simulink model "CryoDetHcd"  (R2016b)
settings: Solver=ode45  StartTime=0.0  StopTime=1e-3  RelTol=1e-3
PreLoadFcn:
  | setup_hcd
values from neighbouring files (symbols this model uses):
  A = sqrt(0.5*erfc(x))    [setup_hcd.m]
  etaRomData = zeros(1,128)    [setup_hcd.m]
  Fadc = 614e6    (= 614000000)    [setup_hcd.m]
  freqRomData = zeros(1,128)    [setup_hcd.m]
  freqRomData1 = zeros(1,128)    [setup_hcd.m]
  freqRomData2 = zeros(1,128)    [setup_hcd.m]
  freqRomData3 = zeros(1,128)    [setup_hcd.m]
undefined symbols (not defined in the file or in its folder): AXI4, B, C, D, j, Lite
libraries: xbsIndex_r4 x2151, CryoDetLibCMB x28, hdlsllib x8, dspsigops x2, simulink x1
(part 6 of 17)

== system CryoDetHcd/DspCore/DSP/analysis_pipelined/Analysis0/channel_select1 ==
  tready : Inport
  data_valid : Inport  Port=2
  Constant : xbsIndex_r4/Constant  const=6  gui_display_data_type=Fixed-point  arith_type=Unsigned  n_bits=3  bin_pt=0  preci_type=Single  exp_width=8  frac_width=24  explicit_period=off  period=1  equ=P=C  opselect=C  inp2=PCIN>>17  opr=+  inp1=P  carry=CIN  dbl_ovrd=off  block_type=constant
  Counter : xbsIndex_r4/Counter  cnt_type=Free Running  cnt_to=Inf  operation=Up  start_count=0  cnt_by_val=1  arith_type=Unsigned  n_bits=3  bin_pt=0  load_pin=off  rst=on  en=on  explicit_period=on  period=2/Fadc  use_behavioral_HDL=off  implementation=Fabric  dbl_ovrd=off  block_type=counter
  Logical6 : xbsIndex_r4/Logical  logical_function=AND  inputs=2  en=off  latency=1  precision=Full  arith_type=Unsigned  n_bits=16  bin_pt=0  align_bp=on  dbl_ovrd=off  block_type=logical
  Relational : xbsIndex_r4/Relational  mode=a=b  op_type=Bool  en=off  latency=1  dbl_ovrd=off  block_type=relational
  tvalid : Outport
  tdata_fsel : Outport  Port=2
  t_last : Outport  Port=3
  wires:
  Logical6/1 -> Counter/2, tvalid/1
  data_valid/1 -> Logical6/2
  Counter/1 -> Relational/2, tdata_fsel/1
  tready/1 -> Logical6/1
  Relational/1 -> t_last/1
  Constant/1 -> Relational/1
  [reset] -> Counter/1

== system CryoDetHcd/DspCore/DSP/analysis_pipelined/Analysis0/scale1 ==
  note: do we saturate here or later???
  sel : Inport
  valid_i : Inport  Port=2
  In1 : Inport  Port=3
  Convert2 : xbsIndex_r4/Convert  gui_display_data_type=Boolean  arith_type=Boolean  n_bits=16  bin_pt=15  float_type=Single  exp_bits=8  fraction_bits=24  quantization=Truncate  overflow=Flag as error  en=off  latency=0  pipeline=off  dbl_ovrd=off  block_type=convert
  Delay : xbsIndex_r4/Delay  rst=off  infoeditControl=Selection of Reset will increase slice count due to use of real FFs and instead of SRLs  en=off  latency=1  reg_retiming=off  dbl_ovrd=off  block_type=delay
  Delay1 : xbsIndex_r4/Delay  rst=off  infoeditControl=Selection of Reset will increase slice count due to use of real FFs and instead of SRLs  en=off  latency=1  reg_retiming=off  dbl_ovrd=off  block_type=delay
  Delay2 : xbsIndex_r4/Delay  rst=off  infoeditControl=Selection of Reset will increase slice count due to use of real FFs and instead of SRLs  en=off  latency=1  reg_retiming=off  dbl_ovrd=off  block_type=delay
  Mux1 : xbsIndex_r4/Mux  inputs=2  en=off  latency=1  precision=User Defined  arith_type="Signed  (2's comp)"  n_bits=18  bin_pt=17  quantization=Truncate  overflow=Saturate  dbl_ovrd=off  block_type=mux
  Mux2 : xbsIndex_r4/Mux  inputs=2  en=off  latency=1  precision=User Defined  arith_type="Signed  (2's comp)"  n_bits=18  bin_pt=17  quantization=Truncate  overflow=Saturate  dbl_ovrd=off  block_type=mux
  high : xbsIndex_r4/BitBasher  bitexpr=|  display_expr=off  sr_1=im_out  arith_type1="Signed  (2's comp)"  bin_pt1=17  sr_2=re_out  arith_type2="Signed  (2's comp)"  bin_pt2=17  sr_3=indx  arith_type3=Unsigned  bin_pt3=0  sr_4=tlast  arith_type4=Unsigned  bin_pt4=0  dbl_ovrd=off  block_type=bitbasher
      | im_out ={ in[39:21] }
      | re_out = { in[18:0] }
      | indx    = { in[44:42] } 
      | tlast     = { in[45] }
  slice8 : xbsIndex_r4/BitBasher  bitexpr=|  display_expr=off  sr_1=im_out  arith_type1="Signed  (2's comp)"  bin_pt1=17  sr_2=re_out  arith_type2="Signed  (2's comp)"  bin_pt2=17  sr_3=indx  arith_type3=Unsigned  bin_pt3=0  sr_4=tlast  arith_type4=Unsigned  bin_pt4=0  dbl_ovrd=off  block_type=bitbasher
      | im_out ={ in[39:22] }
      | re_out = { in[18:1] }
      | indx    = { in[44:42] } 
      | tlast     = { in[45] }
  valid_o : Outport
  im : Outport  Port=2
  re : Outport  Port=3
  indx : Outport  Port=4
  tlast : Outport  Port=5
  wires:
  Convert2/1 -> Delay2/1
  In1/1 -> slice8/1, high/1
  high/3 -> Delay1/1
  high/4 -> Convert2/1
  high/2 -> Mux1/3
  slice8/2 -> Mux1/2
  Mux1/1 -> re/1
  high/1 -> Mux2/3
  Delay2/1 -> tlast/1
  valid_i/1 -> Delay/1
  slice8/1 -> Mux2/2
  Delay/1 -> valid_o/1
  Mux2/1 -> im/1
  Delay1/1 -> indx/1
  sel/1 -> Mux2/1, Mux1/1

== system CryoDetHcd/DspCore/DSP/analysis_pipelined/Analysis0/scale2 ==
  note: do we saturate here or later???
  sel : Inport
  valid_i : Inport  Port=2
  In1 : Inport  Port=3
  Delay : xbsIndex_r4/Delay  rst=off  infoeditControl=Selection of Reset will increase slice count due to use of real FFs and instead of SRLs  en=off  latency=1  reg_retiming=off  dbl_ovrd=off  block_type=delay
  Delay1 : xbsIndex_r4/Delay  rst=off  infoeditControl=Selection of Reset will increase slice count due to use of real FFs and instead of SRLs  en=off  latency=1  reg_retiming=off  dbl_ovrd=off  block_type=delay
  Mux1 : xbsIndex_r4/Mux  inputs=2  en=off  latency=1  precision=User Defined  arith_type="Signed  (2's comp)"  n_bits=18  bin_pt=17  quantization=Truncate  overflow=Saturate  dbl_ovrd=off  block_type=mux
  Mux2 : xbsIndex_r4/Mux  inputs=2  en=off  latency=1  precision=User Defined  arith_type="Signed  (2's comp)"  n_bits=18  bin_pt=17  quantization=Truncate  overflow=Saturate  dbl_ovrd=off  block_type=mux
  high : xbsIndex_r4/BitBasher  bitexpr=|  display_expr=off  sr_1=re  arith_type1="Signed  (2's comp)"  bin_pt1=17  sr_2=im  arith_type2="Signed  (2's comp)"  bin_pt2=17  sr_3=indx  arith_type3=Unsigned  bin_pt3=0  sr_4=4  arith_type4=Unsigned  bin_pt4=0  dbl_ovrd=off  block_type=bitbasher
      | re={in[18:0]}
      | im={in[44:26]}
      | indx ={in[54:52]}
  nominal : xbsIndex_r4/BitBasher  bitexpr=|  display_expr=off  sr_1=re  arith_type1="Signed  (2's comp)"  bin_pt1=17  sr_2=im  arith_type2="Signed  (2's comp)"  bin_pt2=17  sr_3=indx  arith_type3=Unsigned  bin_pt3=0  sr_4=4  arith_type4=Unsigned  bin_pt4=0  dbl_ovrd=off  block_type=bitbasher
      | re={in[18:1]}
      | im={in[44:27]}
      | indx ={in[54:52]}
  valid_o : Outport
  re : Outport  Port=2
  im : Outport  Port=3
  indx : Outport  Port=4
  wires:
  sel/1 -> Mux1/1, Mux2/1
  Delay1/1 -> indx/1
  Delay/1 -> valid_o/1
  valid_i/1 -> Delay/1
  In1/1 -> nominal/1, high/1
  Mux2/1 -> re/1
  Mux1/1 -> im/1
  high/3 -> Delay1/1
  high/2 -> Mux1/3
  high/1 -> Mux2/3
  nominal/1 -> Mux2/2
  nominal/2 -> Mux1/2

== system CryoDetHcd/DspCore/DSP/analysis_pipelined/Analysis0/scale3 ==
  note: do we saturate here or later???
  sel : Inport
  valid_i : Inport  Port=2
  In1 : Inport  Port=3
  Delay : xbsIndex_r4/Delay  rst=off  infoeditControl=Selection of Reset will increase slice count due to use of real FFs and instead of SRLs  en=off  latency=1  reg_retiming=off  dbl_ovrd=off  block_type=delay
  Delay1 : xbsIndex_r4/Delay  rst=off  infoeditControl=Selection of Reset will increase slice count due to use of real FFs and instead of SRLs  en=off  latency=1  reg_retiming=off  dbl_ovrd=off  block_type=delay
  Mux1 : xbsIndex_r4/Mux  inputs=2  en=off  latency=1  precision=User Defined  arith_type="Signed  (2's comp)"  n_bits=18  bin_pt=17  quantization=Truncate  overflow=Saturate  dbl_ovrd=off  block_type=mux
  Mux2 : xbsIndex_r4/Mux  inputs=2  en=off  latency=1  precision=User Defined  arith_type="Signed  (2's comp)"  n_bits=18  bin_pt=17  quantization=Truncate  overflow=Saturate  dbl_ovrd=off  block_type=mux
  high : xbsIndex_r4/BitBasher  bitexpr=|  display_expr=off  sr_1=re  arith_type1="Signed  (2's comp)"  bin_pt1=17  sr_2=im  arith_type2="Signed  (2's comp)"  bin_pt2=17  sr_3=indx  arith_type3=Unsigned  bin_pt3=0  sr_4=4  arith_type4=Unsigned  bin_pt4=0  dbl_ovrd=off  block_type=bitbasher
      | re={in[18:0]}
      | im={in[44:26]}
      | indx ={in[54:52]}
  nominal : xbsIndex_r4/BitBasher  bitexpr=|  display_expr=off  sr_1=re  arith_type1="Signed  (2's comp)"  bin_pt1=17  sr_2=im  arith_type2="Signed  (2's comp)"  bin_pt2=17  sr_3=indx  arith_type3=Unsigned  bin_pt3=0  sr_4=4  arith_type4=Unsigned  bin_pt4=0  dbl_ovrd=off  block_type=bitbasher
      | re={in[18:1]}
      | im={in[44:27]}
      | indx ={in[54:52]}
  valid_o : Outport
  re : Outport  Port=2
  im : Outport  Port=3
  indx : Outport  Port=4
  wires:
  nominal/2 -> Mux1/2
  nominal/1 -> Mux2/2
  high/1 -> Mux2/3
  high/2 -> Mux1/3
  high/3 -> Delay1/1
  Mux1/1 -> im/1
  Mux2/1 -> re/1
  In1/1 -> high/1, nominal/1
  valid_i/1 -> Delay/1
  Delay/1 -> valid_o/1
  Delay1/1 -> indx/1
  sel/1 -> Mux2/1, Mux1/1

== system CryoDetHcd/DspCore/DSP/analysis_pipelined/Analysis0/scale4 ==
  note: do we saturate here or later???
  sel : Inport
  valid_i : Inport  Port=2
  In1 : Inport  Port=3
  Convert2 : xbsIndex_r4/Convert  gui_display_data_type=Boolean  arith_type=Boolean  n_bits=16  bin_pt=15  float_type=Single  exp_bits=8  fraction_bits=24  quantization=Truncate  overflow=Flag as error  en=off  latency=0  pipeline=off  dbl_ovrd=off  block_type=convert
  Delay : xbsIndex_r4/Delay  rst=off  infoeditControl=Selection of Reset will increase slice count due to use of real FFs and instead of SRLs  en=off  latency=1  reg_retiming=off  dbl_ovrd=off  block_type=delay
  Delay1 : xbsIndex_r4/Delay  rst=off  infoeditControl=Selection of Reset will increase slice count due to use of real FFs and instead of SRLs  en=off  latency=1  reg_retiming=off  dbl_ovrd=off  block_type=delay
  Delay2 : xbsIndex_r4/Delay  rst=off  infoeditControl=Selection of Reset will increase slice count due to use of real FFs and instead of SRLs  en=off  latency=1  reg_retiming=off  dbl_ovrd=off  block_type=delay
  Mux1 : xbsIndex_r4/Mux  inputs=2  en=off  latency=1  precision=User Defined  arith_type="Signed  (2's comp)"  n_bits=18  bin_pt=17  quantization=Truncate  overflow=Saturate  dbl_ovrd=off  block_type=mux
  Mux2 : xbsIndex_r4/Mux  inputs=2  en=off  latency=1  precision=User Defined  arith_type="Signed  (2's comp)"  n_bits=18  bin_pt=17  quantization=Truncate  overflow=Saturate  dbl_ovrd=off  block_type=mux
  high : xbsIndex_r4/BitBasher  bitexpr=|  display_expr=off  sr_1=im_out  arith_type1="Signed  (2's comp)"  bin_pt1=17  sr_2=re_out  arith_type2="Signed  (2's comp)"  bin_pt2=17  sr_3=indx  arith_type3=Unsigned  bin_pt3=0  sr_4=tlast  arith_type4=Unsigned  bin_pt4=0  dbl_ovrd=off  block_type=bitbasher
      | im_out ={ in[39:21] }
      | re_out = { in[18:0] }
      | indx    = { in[44:42] } 
      | tlast     = { in[45] }
  slice8 : xbsIndex_r4/BitBasher  bitexpr=|  display_expr=off  sr_1=im_out  arith_type1="Signed  (2's comp)"  bin_pt1=17  sr_2=re_out  arith_type2="Signed  (2's comp)"  bin_pt2=17  sr_3=indx  arith_type3=Unsigned  bin_pt3=0  sr_4=tlast  arith_type4=Unsigned  bin_pt4=0  dbl_ovrd=off  block_type=bitbasher
      | im_out ={ in[39:22] }
      | re_out = { in[18:1] }
      | indx    = { in[44:42] } 
      | tlast     = { in[45] }
  valid_o : Outport
  im : Outport  Port=2
  re : Outport  Port=3
  indx : Outport  Port=4
  tlast : Outport  Port=5
  wires:
  sel/1 -> Mux1/1, Mux2/1
  Delay1/1 -> indx/1
  Mux2/1 -> im/1
  Delay/1 -> valid_o/1
  slice8/1 -> Mux2/2
  valid_i/1 -> Delay/1
  Delay2/1 -> tlast/1
  high/1 -> Mux2/3
  Mux1/1 -> re/1
  slice8/2 -> Mux1/2
  high/2 -> Mux1/3
  high/4 -> Convert2/1
  high/3 -> Delay1/1
  In1/1 -> high/1, slice8/1
  Convert2/1 -> Delay2/1

== system CryoDetHcd/DspCore/DSP/analysis_pipelined/Analysis1/channel_select1 ==
  tready : Inport
  data_valid : Inport  Port=2
  Constant : xbsIndex_r4/Constant  const=6  gui_display_data_type=Fixed-point  arith_type=Unsigned  n_bits=3  bin_pt=0  preci_type=Single  exp_width=8  frac_width=24  explicit_period=off  period=1  equ=P=C  opselect=C  inp2=PCIN>>17  opr=+  inp1=P  carry=CIN  dbl_ovrd=off  block_type=constant
  Counter : xbsIndex_r4/Counter  cnt_type=Free Running  cnt_to=Inf  operation=Up  start_count=0  cnt_by_val=1  arith_type=Unsigned  n_bits=3  bin_pt=0  load_pin=off  rst=on  en=on  explicit_period=on  period=2/Fadc  use_behavioral_HDL=off  implementation=Fabric  dbl_ovrd=off  block_type=counter
  Logical6 : xbsIndex_r4/Logical  logical_function=AND  inputs=2  en=off  latency=1  precision=Full  arith_type=Unsigned  n_bits=16  bin_pt=0  align_bp=on  dbl_ovrd=off  block_type=logical
  Relational : xbsIndex_r4/Relational  mode=a=b  op_type=Bool  en=off  latency=1  dbl_ovrd=off  block_type=relational
  tvalid : Outport
  tdata_fsel : Outport  Port=2
  t_last : Outport  Port=3
  wires:
  [reset] -> Counter/1
  Constant/1 -> Relational/1
  Relational/1 -> t_last/1
  tready/1 -> Logical6/1
  Counter/1 -> tdata_fsel/1, Relational/2
  data_valid/1 -> Logical6/2
  Logical6/1 -> tvalid/1, Counter/2

== system CryoDetHcd/DspCore/DSP/analysis_pipelined/Analysis1/scale1 ==
  note: do we saturate here or later???
  sel : Inport
  valid_i : Inport  Port=2
  In1 : Inport  Port=3
  Convert2 : xbsIndex_r4/Convert  gui_display_data_type=Boolean  arith_type=Boolean  n_bits=16  bin_pt=15  float_type=Single  exp_bits=8  fraction_bits=24  quantization=Truncate  overflow=Flag as error  en=off  latency=0  pipeline=off  dbl_ovrd=off  block_type=convert
  Delay : xbsIndex_r4/Delay  rst=off  infoeditControl=Selection of Reset will increase slice count due to use of real FFs and instead of SRLs  en=off  latency=1  reg_retiming=off  dbl_ovrd=off  block_type=delay
  Delay1 : xbsIndex_r4/Delay  rst=off  infoeditControl=Selection of Reset will increase slice count due to use of real FFs and instead of SRLs  en=off  latency=1  reg_retiming=off  dbl_ovrd=off  block_type=delay
  Delay2 : xbsIndex_r4/Delay  rst=off  infoeditControl=Selection of Reset will increase slice count due to use of real FFs and instead of SRLs  en=off  latency=1  reg_retiming=off  dbl_ovrd=off  block_type=delay
  Mux1 : xbsIndex_r4/Mux  inputs=2  en=off  latency=1  precision=User Defined  arith_type="Signed  (2's comp)"  n_bits=18  bin_pt=17  quantization=Truncate  overflow=Saturate  dbl_ovrd=off  block_type=mux
  Mux2 : xbsIndex_r4/Mux  inputs=2  en=off  latency=1  precision=User Defined  arith_type="Signed  (2's comp)"  n_bits=18  bin_pt=17  quantization=Truncate  overflow=Saturate  dbl_ovrd=off  block_type=mux
  high : xbsIndex_r4/BitBasher  bitexpr=|  display_expr=off  sr_1=im_out  arith_type1="Signed  (2's comp)"  bin_pt1=17  sr_2=re_out  arith_type2="Signed  (2's comp)"  bin_pt2=17  sr_3=indx  arith_type3=Unsigned  bin_pt3=0  sr_4=tlast  arith_type4=Unsigned  bin_pt4=0  dbl_ovrd=off  block_type=bitbasher
      | im_out ={ in[39:21] }
      | re_out = { in[18:0] }
      | indx    = { in[44:42] } 
      | tlast     = { in[45] }
  slice8 : xbsIndex_r4/BitBasher  bitexpr=|  display_expr=off  sr_1=im_out  arith_type1="Signed  (2's comp)"  bin_pt1=17  sr_2=re_out  arith_type2="Signed  (2's comp)"  bin_pt2=17  sr_3=indx  arith_type3=Unsigned  bin_pt3=0  sr_4=tlast  arith_type4=Unsigned  bin_pt4=0  dbl_ovrd=off  block_type=bitbasher
      | im_out ={ in[39:22] }
      | re_out = { in[18:1] }
      | indx    = { in[44:42] } 
      | tlast     = { in[45] }
  valid_o : Outport
  im : Outport  Port=2
  re : Outport  Port=3
  indx : Outport  Port=4
  tlast : Outport  Port=5
  wires:
  sel/1 -> Mux1/1, Mux2/1
  Delay1/1 -> indx/1
  Mux2/1 -> im/1
  Delay/1 -> valid_o/1
  slice8/1 -> Mux2/2
  valid_i/1 -> Delay/1
  Delay2/1 -> tlast/1
  high/1 -> Mux2/3
  Mux1/1 -> re/1
  slice8/2 -> Mux1/2
  high/2 -> Mux1/3
  high/4 -> Convert2/1
  high/3 -> Delay1/1
  In1/1 -> high/1, slice8/1
  Convert2/1 -> Delay2/1

== system CryoDetHcd/DspCore/DSP/analysis_pipelined/Analysis1/scale2 ==
  note: do we saturate here or later???
  sel : Inport
  valid_i : Inport  Port=2
  In1 : Inport  Port=3
  Delay : xbsIndex_r4/Delay  rst=off  infoeditControl=Selection of Reset will increase slice count due to use of real FFs and instead of SRLs  en=off  latency=1  reg_retiming=off  dbl_ovrd=off  block_type=delay
  Delay1 : xbsIndex_r4/Delay  rst=off  infoeditControl=Selection of Reset will increase slice count due to use of real FFs and instead of SRLs  en=off  latency=1  reg_retiming=off  dbl_ovrd=off  block_type=delay
  Mux1 : xbsIndex_r4/Mux  inputs=2  en=off  latency=1  precision=User Defined  arith_type="Signed  (2's comp)"  n_bits=18  bin_pt=17  quantization=Truncate  overflow=Saturate  dbl_ovrd=off  block_type=mux
  Mux2 : xbsIndex_r4/Mux  inputs=2  en=off  latency=1  precision=User Defined  arith_type="Signed  (2's comp)"  n_bits=18  bin_pt=17  quantization=Truncate  overflow=Saturate  dbl_ovrd=off  block_type=mux
  high : xbsIndex_r4/BitBasher  bitexpr=|  display_expr=off  sr_1=re  arith_type1="Signed  (2's comp)"  bin_pt1=17  sr_2=im  arith_type2="Signed  (2's comp)"  bin_pt2=17  sr_3=indx  arith_type3=Unsigned  bin_pt3=0  sr_4=4  arith_type4=Unsigned  bin_pt4=0  dbl_ovrd=off  block_type=bitbasher
      | re={in[18:0]}
      | im={in[44:26]}
      | indx ={in[54:52]}
  nominal : xbsIndex_r4/BitBasher  bitexpr=|  display_expr=off  sr_1=re  arith_type1="Signed  (2's comp)"  bin_pt1=17  sr_2=im  arith_type2="Signed  (2's comp)"  bin_pt2=17  sr_3=indx  arith_type3=Unsigned  bin_pt3=0  sr_4=4  arith_type4=Unsigned  bin_pt4=0  dbl_ovrd=off  block_type=bitbasher
      | re={in[18:1]}
      | im={in[44:27]}
      | indx ={in[54:52]}
  valid_o : Outport
  re : Outport  Port=2
  im : Outport  Port=3
  indx : Outport  Port=4
  wires:
  nominal/2 -> Mux1/2
  nominal/1 -> Mux2/2
  high/1 -> Mux2/3
  high/2 -> Mux1/3
  high/3 -> Delay1/1
  Mux1/1 -> im/1
  Mux2/1 -> re/1
  In1/1 -> high/1, nominal/1
  valid_i/1 -> Delay/1
  Delay/1 -> valid_o/1
  Delay1/1 -> indx/1
  sel/1 -> Mux2/1, Mux1/1

== system CryoDetHcd/DspCore/DSP/analysis_pipelined/Analysis1/scale3 ==
  note: do we saturate here or later???
  sel : Inport
  valid_i : Inport  Port=2
  In1 : Inport  Port=3
  Delay : xbsIndex_r4/Delay  rst=off  infoeditControl=Selection of Reset will increase slice count due to use of real FFs and instead of SRLs  en=off  latency=1  reg_retiming=off  dbl_ovrd=off  block_type=delay
  Delay1 : xbsIndex_r4/Delay  rst=off  infoeditControl=Selection of Reset will increase slice count due to use of real FFs and instead of SRLs  en=off  latency=1  reg_retiming=off  dbl_ovrd=off  block_type=delay
  Mux1 : xbsIndex_r4/Mux  inputs=2  en=off  latency=1  precision=User Defined  arith_type="Signed  (2's comp)"  n_bits=18  bin_pt=17  quantization=Truncate  overflow=Saturate  dbl_ovrd=off  block_type=mux
  Mux2 : xbsIndex_r4/Mux  inputs=2  en=off  latency=1  precision=User Defined  arith_type="Signed  (2's comp)"  n_bits=18  bin_pt=17  quantization=Truncate  overflow=Saturate  dbl_ovrd=off  block_type=mux
  high : xbsIndex_r4/BitBasher  bitexpr=|  display_expr=off  sr_1=re  arith_type1="Signed  (2's comp)"  bin_pt1=17  sr_2=im  arith_type2="Signed  (2's comp)"  bin_pt2=17  sr_3=indx  arith_type3=Unsigned  bin_pt3=0  sr_4=4  arith_type4=Unsigned  bin_pt4=0  dbl_ovrd=off  block_type=bitbasher
      | re={in[18:0]}
      | im={in[44:26]}
      | indx ={in[54:52]}
  nominal : xbsIndex_r4/BitBasher  bitexpr=|  display_expr=off  sr_1=re  arith_type1="Signed  (2's comp)"  bin_pt1=17  sr_2=im  arith_type2="Signed  (2's comp)"  bin_pt2=17  sr_3=indx  arith_type3=Unsigned  bin_pt3=0  sr_4=4  arith_type4=Unsigned  bin_pt4=0  dbl_ovrd=off  block_type=bitbasher
      | re={in[18:1]}
      | im={in[44:27]}
      | indx ={in[54:52]}
  valid_o : Outport
  re : Outport  Port=2
  im : Outport  Port=3
  indx : Outport  Port=4
  wires:
  sel/1 -> Mux1/1, Mux2/1
  Delay1/1 -> indx/1
  Delay/1 -> valid_o/1
  valid_i/1 -> Delay/1
  In1/1 -> nominal/1, high/1
  Mux2/1 -> re/1
  Mux1/1 -> im/1
  high/3 -> Delay1/1
  high/2 -> Mux1/3
  high/1 -> Mux2/3
  nominal/1 -> Mux2/2
  nominal/2 -> Mux1/2

== system CryoDetHcd/DspCore/DSP/analysis_pipelined/Analysis1/scale4 ==
  note: do we saturate here or later???
  sel : Inport
  valid_i : Inport  Port=2
  In1 : Inport  Port=3
  Convert2 : xbsIndex_r4/Convert  gui_display_data_type=Boolean  arith_type=Boolean  n_bits=16  bin_pt=15  float_type=Single  exp_bits=8  fraction_bits=24  quantization=Truncate  overflow=Flag as error  en=off  latency=0  pipeline=off  dbl_ovrd=off  block_type=convert
  Delay : xbsIndex_r4/Delay  rst=off  infoeditControl=Selection of Reset will increase slice count due to use of real FFs and instead of SRLs  en=off  latency=1  reg_retiming=off  dbl_ovrd=off  block_type=delay
  Delay1 : xbsIndex_r4/Delay  rst=off  infoeditControl=Selection of Reset will increase slice count due to use of real FFs and instead of SRLs  en=off  latency=1  reg_retiming=off  dbl_ovrd=off  block_type=delay
  Delay2 : xbsIndex_r4/Delay  rst=off  infoeditControl=Selection of Reset will increase slice count due to use of real FFs and instead of SRLs  en=off  latency=1  reg_retiming=off  dbl_ovrd=off  block_type=delay
  Mux1 : xbsIndex_r4/Mux  inputs=2  en=off  latency=1  precision=User Defined  arith_type="Signed  (2's comp)"  n_bits=18  bin_pt=17  quantization=Truncate  overflow=Saturate  dbl_ovrd=off  block_type=mux
  Mux2 : xbsIndex_r4/Mux  inputs=2  en=off  latency=1  precision=User Defined  arith_type="Signed  (2's comp)"  n_bits=18  bin_pt=17  quantization=Truncate  overflow=Saturate  dbl_ovrd=off  block_type=mux
  high : xbsIndex_r4/BitBasher  bitexpr=|  display_expr=off  sr_1=im_out  arith_type1="Signed  (2's comp)"  bin_pt1=17  sr_2=re_out  arith_type2="Signed  (2's comp)"  bin_pt2=17  sr_3=indx  arith_type3=Unsigned  bin_pt3=0  sr_4=tlast  arith_type4=Unsigned  bin_pt4=0  dbl_ovrd=off  block_type=bitbasher
      | im_out ={ in[39:21] }
      | re_out = { in[18:0] }
      | indx    = { in[44:42] } 
      | tlast     = { in[45] }
  slice8 : xbsIndex_r4/BitBasher  bitexpr=|  display_expr=off  sr_1=im_out  arith_type1="Signed  (2's comp)"  bin_pt1=17  sr_2=re_out  arith_type2="Signed  (2's comp)"  bin_pt2=17  sr_3=indx  arith_type3=Unsigned  bin_pt3=0  sr_4=tlast  arith_type4=Unsigned  bin_pt4=0  dbl_ovrd=off  block_type=bitbasher
      | im_out ={ in[39:22] }
      | re_out = { in[18:1] }
      | indx    = { in[44:42] } 
      | tlast     = { in[45] }
  valid_o : Outport
  im : Outport  Port=2
  re : Outport  Port=3
  indx : Outport  Port=4
  tlast : Outport  Port=5
  wires:
  Convert2/1 -> Delay2/1
  In1/1 -> slice8/1, high/1
  high/3 -> Delay1/1
  high/4 -> Convert2/1
  high/2 -> Mux1/3
  slice8/2 -> Mux1/2
  Mux1/1 -> re/1
  high/1 -> Mux2/3
  Delay2/1 -> tlast/1
  valid_i/1 -> Delay/1
  slice8/1 -> Mux2/2
  Delay/1 -> valid_o/1
  Mux2/1 -> im/1
  Delay1/1 -> indx/1
  sel/1 -> Mux2/1, Mux1/1

== system CryoDetHcd/DspCore/DSP/channel_processor/channel_processor_x1/Enabled Subsystem ==
  In1 : Inport
  In2 : Inport  Port=2
  Enable : EnablePort
  Buffer : Buffer  N=8  TreatMby1Signals=One channel  OutputFrames=off
  Buffer1 : Buffer  N=8  TreatMby1Signals=One channel  OutputFrames=off
  Out1 : Outport
  Out2 : Outport  Port=2
  wires:
  In1/1 -> Buffer/1
  Buffer/1 -> Out1/1
  In2/1 -> Buffer1/1
  Buffer1/1 -> Out2/1

== system CryoDetHcd/DspCore/DSP/channel_processor/channel_processor_x1/IQ_status_sel ==
  sel : Inport
  Q : Inport  Port=2
  I : Inport  Port=3
  ch : Inport  Port=4
  BitBasher : xbsIndex_r4/BitBasher  bitexpr=out = {I,Q}  display_expr=off  sr_1=out  arith_type1=Unsigned  bin_pt1=0  sr_2=2  arith_type2=Unsigned  bin_pt2=0  sr_3=3  arith_type3=Unsigned  bin_pt3=0  sr_4=4  arith_type4=Unsigned  bin_pt4=0  dbl_ovrd=off  block_type=bitbasher
  Convert : xbsIndex_r4/Convert  gui_display_data_type=Fixed-point  arith_type="Signed  (2's comp)"  n_bits=16  bin_pt=15  float_type=Single  exp_bits=8  fraction_bits=24  quantization=Truncate  overflow=Wrap  en=off  latency=1  pipeline=off  dbl_ovrd=off  block_type=convert
  Convert1 : xbsIndex_r4/Convert  gui_display_data_type=Fixed-point  arith_type="Signed  (2's comp)"  n_bits=16  bin_pt=15  float_type=Single  exp_bits=8  fraction_bits=24  quantization=Truncate  overflow=Wrap  en=off  latency=1  pipeline=off  dbl_ovrd=off  block_type=convert
  Register2 : xbsIndex_r4/Register  init=0  rst=off  en=on  dbl_ovrd=off  block_type=register
  Relational : xbsIndex_r4/Relational  mode=a=b  op_type=Bool  en=off  latency=1  dbl_ovrd=off  block_type=relational
  IQ_status_r : Outport
  wires:
  I/1 -> Convert1/1
  Q/1 -> Convert/1
  Convert1/1 -> BitBasher/2
  ch/1 -> Relational/2
  sel/1 -> Relational/1
  Convert/1 -> BitBasher/1
  BitBasher/1 -> Register2/1
  Register2/1 -> IQ_status_r/1
  Relational/1 -> Register2/2

== system CryoDetHcd/DspCore/DSP/channel_processor/channel_processor_x1/config2_r ==
  In1 : Inport
  BitBasher : xbsIndex_r4/BitBasher  bitexpr=|  display_expr=off  sr_1=ref_delay  arith_type1=Unsigned  bin_pt1=0  sr_2=tone_scale_sel  arith_type2=Unsigned  bin_pt2=0  sr_3=fb_enable  arith_type3=Unsigned  bin_pt3=0  sr_4=fb_polarity  arith_type4=Unsigned  bin_pt4=0  dbl_ovrd=off  block_type=bitbasher
      | ref_delay = {in[2:0]}
      | tone_scale_sel = {in[4:3]}
      | fb_enable = {in[5]}
      | fb_polarity = {in[6]}
  BitBasher1 : xbsIndex_r4/BitBasher  bitexpr=|  display_expr=off  sr_1=iq_swap_sel  arith_type1=Unsigned  bin_pt1=0  sr_2=iq_band_sel  arith_type2=Unsigned  bin_pt2=0  sr_3=iq_ch_sel  arith_type3=Unsigned  bin_pt3=0  sr_4=analysis_iq_ch_sel  arith_type4=Unsigned  bin_pt4=0  dbl_ovrd=off  block_type=bitbasher
      | iq_swap_sel = {in[7]}
      | iq_band_sel = {in[16:15]}
      | iq_ch_sel = {in[14:8]}
      | analysis_iq_ch_sel={in[17:15]}
  ref_delay : Outport
  tone_scale_sel : Outport  Port=2
  fb_enable : Outport  Port=3
  fb_polarity : Outport  Port=4
  iq_swap_sel : Outport  Port=5
  iq_band_sel : Outport  Port=6
  iq_ch_sel : Outport  Port=7
  analysis_iq_sel : Outport  Port=8
  wires:
  BitBasher1/3 -> iq_ch_sel/1
  BitBasher1/2 -> iq_band_sel/1
  BitBasher1/1 -> iq_swap_sel/1
  BitBasher/4 -> fb_polarity/1
  BitBasher/3 -> fb_enable/1
  BitBasher/2 -> tone_scale_sel/1
  BitBasher/1 -> ref_delay/1
  In1/1 -> BitBasher/1, BitBasher1/1
  BitBasher1/4 -> analysis_iq_sel/1

== system CryoDetHcd/DspCore/DSP/channel_processor/channel_processor_x1/config3_r1 ==
  In1 : Inport
  BitBasher1 : xbsIndex_r4/BitBasher  bitexpr=|  display_expr=off  sr_1=fb_gain  arith_type1=Unsigned  bin_pt1=14  sr_2=fb_limit  arith_type2=Unsigned  bin_pt2=16  sr_3=ref_delay  arith_type3=Unsigned  bin_pt3=0  sr_4=4  arith_type4=Unsigned  bin_pt4=0  dbl_ovrd=off  block_type=bitbasher
      | fb_gain = {in[15:0]}
      | fb_limit = {in[31:16]}
  Negate : xbsIndex_r4/Negate  precision=User Defined  arith_type=Unsigned  n_bits=16  bin_pt=15  quantization=Truncate  overflow=Wrap  en=off  latency=2  dbl_ovrd=off  block_type=negate
  fb_gain : Outport
  fb_limit_hi : Outport  Port=2
  fb_limit_lo : Outport  Port=3
  wires:
  BitBasher1/2 -> Negate/1, fb_limit_hi/1
  In1/1 -> BitBasher1/1
  BitBasher1/1 -> fb_gain/1
  Negate/1 -> fb_limit_lo/1

== system CryoDetHcd/DspCore/DSP/channel_processor/channel_processor_x1/scale1 ==
  In1 : Inport
  Bit Slice : hdlsllib/HDL Operations/Bit Slice  lidx=15  ridx=0
  Bit Slice1 : hdlsllib/HDL Operations/Bit Slice  lidx=31  ridx=16
  Data Type Conversion : DataTypeConversion  OutDataTypeStr=int16  ConvertRealWorld=Stored Integer (SI)
  Data Type Conversion1 : DataTypeConversion  OutDataTypeStr=int16  ConvertRealWorld=Stored Integer (SI)
  Q : Outport
  I : Outport  Port=2
  wires:
  In1/1 -> Bit Slice1/1, Bit Slice/1
  Bit Slice/1 -> Data Type Conversion/1
  Data Type Conversion1/1 -> Q/1
  Bit Slice1/1 -> Data Type Conversion1/1
  Data Type Conversion/1 -> I/1

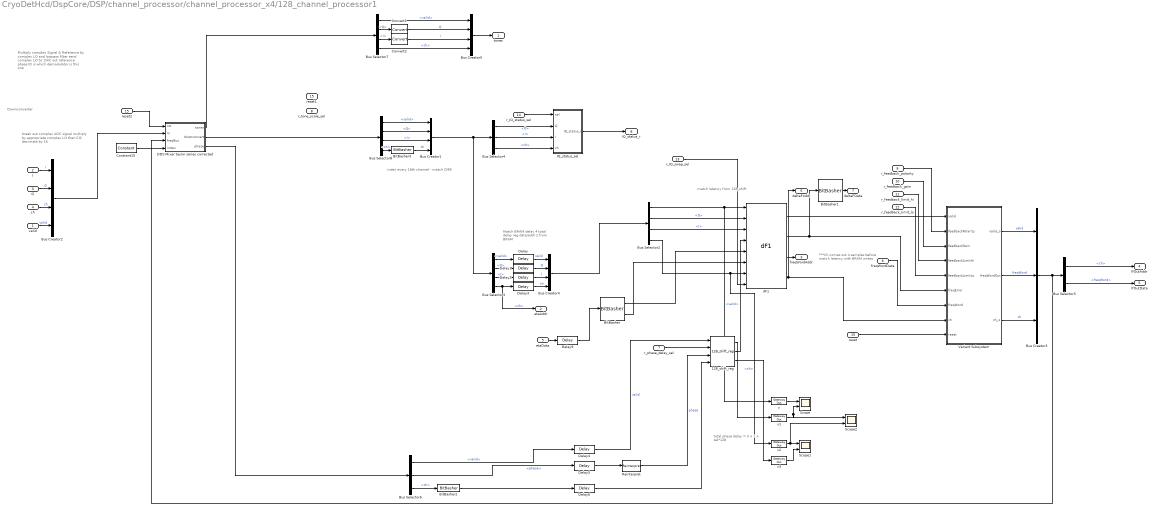
== system CryoDetHcd/DspCore/DSP/channel_processor/channel_processor_x4/128_channel_processor1 ==
  note: ***Ch comes out 4 samples before
      | match latency with BRAM writes
  note: total phase delay =
      | 3 + 1 + sel*128
  note: match latency from 128_shift
  note: Match BRAM delay
      | 4 total delay
      |    reg data/addr
      |    2 from BRAM
  note: break out complex ADC signal
      | multiply by appropriate complex LO
      | then CIC decimate by 16
  note: Multiply complex Signal & Reference
      | by complex LO and lowpass filter
      | send complex LO to:
      | 	DAC out
      | 	reference phase
      | ID is which demodulator is this one
  note: Downconverter
  note: index every 16th channel - match CMB
  valid : Inport
  I : Inport  Port=2
  Q : Inport  Port=3
  ch : Inport  Port=4
  etaData : Inport  Port=5
  freqWordData : Inport  Port=6
  r_phase_delay_sel : Inport  Port=7
  r_tone_scale_sel : Inport  Port=8
  r_feedback_polarity : Inport  Port=9
  r_feedback_gain : Inport  Port=10
  r_feedback_limit_hi : Inport  Port=11
  r_feedback_limit_lo : Inport  Port=12
  r_IQ_swap_sel : Inport  Port=13
  r_IQ_status_sel : Inport  Port=14
  reset : Inport  Port=15
  128_shift_reg : CryoDetLibCMB/128_shift_reg
  BitBasher : xbsIndex_r4/BitBasher  bitexpr=|  display_expr=off  sr_1=etaPhase  arith_type1="Signed  (2's comp)"  bin_pt1=15  sr_2=etaMag  arith_type2="Signed  (2's comp)"  bin_pt2=10  sr_3=3  arith_type3=Unsigned  bin_pt3=0  sr_4=4  arith_type4=Unsigned  bin_pt4=0  dbl_ovrd=off  block_type=bitbasher
      | etaPhase = {in[31:16]}
      | etaMag = {in[15:0]}
  BitBasher1 : xbsIndex_r4/BitBasher  bitexpr=deltaF = {8'b0, in[23:0]}  display_expr=off  sr_1=deltaF  arith_type1="Signed  (2's comp)"  bin_pt1=15  sr_2=etaMag  arith_type2="Signed  (2's comp)"  bin_pt2=10  sr_3=3  arith_type3=Unsigned  bin_pt3=0  sr_4=4  arith_type4=Unsigned  bin_pt4=0  dbl_ovrd=off  block_type=bitbasher
  BitBasher2 : xbsIndex_r4/BitBasher  bitexpr=out = {in, 4'b0000}  display_expr=off  sr_1=out  arith_type1=Unsigned  bin_pt1=0  sr_2=2  arith_type2=Unsigned  bin_pt2=0  sr_3=3  arith_type3=Unsigned  bin_pt3=0  sr_4=4  arith_type4=Unsigned  bin_pt4=0  dbl_ovrd=off  block_type=bitbasher
  BitBasher3 : xbsIndex_r4/BitBasher  bitexpr=out = {in, 4'b0000}  display_expr=off  sr_1=out  arith_type1=Unsigned  bin_pt1=0  sr_2=2  arith_type2=Unsigned  bin_pt2=0  sr_3=3  arith_type3=Unsigned  bin_pt3=0  sr_4=4  arith_type4=Unsigned  bin_pt4=0  dbl_ovrd=off  block_type=bitbasher
  Bus Creator{1..2,4..5} (4 alike) : BusCreator  Inputs=4
  Bus Creator3 : BusCreator  Inputs=3
  Bus Selector{2..3,7..8} (4 alike) : BusSelector  OutputSignals=valid,Q,I,ch
  Bus Selector4 : BusSelector  OutputSignals=Q,I,ch
  Bus Selector5 : BusSelector  OutputSignals=ch,freqWord
  Bus Selector6 : BusSelector  OutputSignals=valid,phase,ch
  Constant15 : xbsIndex_r4/Constant  const=0  gui_display_data_type=Fixed-point  arith_type=Unsigned  n_bits=4  bin_pt=0  preci_type=Single  exp_width=8  frac_width=24  explicit_period=off  period=1  equ=P=C  opselect=C  inp2=PCIN>>17  opr=+  inp1=P  carry=CIN  dbl_ovrd=off  block_type=constant
  Convert1 : xbsIndex_r4/Convert  gui_display_data_type=Fixed-point  arith_type="Signed  (2's comp)"  n_bits=16  bin_pt=15  float_type=Single  exp_bits=8  fraction_bits=24  quantization=Truncate  overflow=Wrap  en=off  latency=0  pipeline=off  dbl_ovrd=off  block_type=convert
  Convert2 : xbsIndex_r4/Convert  gui_display_data_type=Fixed-point  arith_type="Signed  (2's comp)"  n_bits=16  bin_pt=15  float_type=Single  exp_bits=8  fraction_bits=24  quantization=Truncate  overflow=Wrap  en=off  latency=0  pipeline=off  dbl_ovrd=off  block_type=convert
  DDS Mixer taylor series corrected : Subsystem  AncestorBlock=CryoDetLibCMB/DDS Mixer taylor series corrected
  Delay{,1..3} (4 alike) : xbsIndex_r4/Delay  rst=off  infoeditControl=Selection of Reset will increase slice count due to use of real FFs and instead of SRLs  en=off  latency=5  reg_retiming=off  dbl_ovrd=off  block_type=delay
  Delay{4..6,9} (4 alike) : xbsIndex_r4/Delay  rst=off  infoeditControl=Selection of Reset will increase slice count due to use of real FFs and instead of SRLs  en=off  latency=1  reg_retiming=off  dbl_ovrd=off  block_type=delay
  IQ_status_sel : Subsystem
  Reinterpret : xbsIndex_r4/Reinterpret  force_arith_type=on  arith_type="Signed  (2's comp)"  force_bin_pt=on  bin_pt=15  block_type=reinterpret
  Scope : Scope  NumInputPorts=2
  Scope1 : Scope  NumInputPorts=2
  Scope2 : Scope  NumInputPorts=2
  Variant Subsystem : Subsystem  Variant=on  OverrideUsingVariant=Variant1
  dF1 : CryoDetLibCMB/dF1
  reset1 : InportShadow  Port=15
  reset2 : InportShadow  Port=15
  v{,1..3} (4 alike) : xbsIndex_r4/Gateway Out  inherit_from_input=off  hdl_port=off  rows=1  columns=1  UseAsDAC=off  DACChannel='1'  interface=None  automatic_assignment=on  address_offset=hex2dec('00')  intf_name=''  intf_description=''  timing_constraint=None  locs_specified=off  LOCs={}  io_standard={}  block_type=gatewayout
  tones : Outport
  etaAddr : Outport  Port=2
  freqWordAddr : Outport  Port=3
  lfOutAddr : Outport  Port=4
  lfOutData : Outport  Port=5
  deltaFAddr : Outport  Port=6
  deltaFData : Outport  Port=7
  IQ_status_r : Outport  Port=8
  wires:
  v2/1 -> Scope1/1, Scope2/2
  v1/1 -> Scope/2, Scope2/1
  BitBasher2/1 -> Delay6/1
  DDS Mixer taylor series corrected/2(downconvert) -> Bus Selector8/1
  Bus Creator1/1 -> Bus Selector4/1, Bus Selector3/1
  Bus Selector8/3 -> Bus Creator1/3  "<I>"
  Bus Selector8/1 -> Bus Creator1/1  "<valid>"
  Bus Selector8/2 -> Bus Creator1/2  "<Q>"
  BitBasher3/1 -> Bus Creator1/4  "ch"
  Bus Selector8/4 -> BitBasher3/1  "<ch>"
  Bus Selector7/3 -> Convert2/1  "<I>"
  Bus Selector7/2 -> Convert1/1  "<Q>"
  Bus Selector6/3 -> BitBasher2/1  "<ch>"
  DDS Mixer taylor series corrected/3(phase) -> Bus Selector6/1
  Bus Creator3/1 -> Bus Selector5/1, DDS Mixer taylor series corrected/3(freqBus)
  reset2/1 -> DDS Mixer taylor series corrected/1(rst)
  Constant15/1 -> DDS Mixer taylor series corrected/4(index)
  Delay6/1 -> 128_shift_reg/4
  Delay9/1 -> BitBasher/1
  IQ_status_sel/1(IQ_status_r) -> IQ_status_r/1
  r_IQ_status_sel/1 -> IQ_status_sel/1(sel)
  Bus Selector4/3 -> IQ_status_sel/4(ch)  "<ch>"
  Bus Selector4/2 -> IQ_status_sel/3(I)  "<I>"
  Bus Selector4/1 -> IQ_status_sel/2(Q)  "<Q>"
  r_IQ_swap_sel/1 -> dF1/8
  128_shift_reg/3 -> v3/1
  v3/1 -> Scope1/2
  128_shift_reg/1 -> v1/1
  v/1 -> Scope/1
  Bus Creator2/1 -> DDS Mixer taylor series corrected/2(In)
  DDS Mixer taylor series corrected/1(tones) -> Bus Selector7/1
  I/1 -> Bus Creator2/1  "I"
  Q/1 -> Bus Creator2/2  "Q"
  ch/1 -> Bus Creator2/3  "ch"
  valid/1 -> Bus Creator2/4  "valid"
  Delay/1 -> Bus Creator4/1  "valid"
  Delay1/1 -> Bus Creator4/2  "Q"
  Delay2/1 -> Bus Creator4/3  "I"
  Delay3/1 -> Bus Creator4/4  "ch"
  etaData/1 -> Delay9/1
  Bus Creator4/1 -> Bus Selector2/1
  BitBasher1/1 -> deltaFData/1
  Bus Selector3/1 -> Delay/1  "<valid>"
  Bus Selector3/2 -> Delay1/1  "<Q>"
  Bus Selector3/3 -> Delay2/1  "<I>"
  Bus Selector3/4 -> Delay3/1, etaAddr/1  "<ch>"
  Convert2/1 -> Bus Creator5/3  "I"
  Convert1/1 -> Bus Creator5/2  "Q"
  Bus Selector7/4 -> Bus Creator5/4  "<ch>"
  Bus Selector7/1 -> Bus Creator5/1  "<valid>"
  Bus Creator5/1 -> tones/1
  Bus Selector2/1 -> dF1/1, v/1  "<valid>"
  Bus Selector2/2 -> dF1/2  "<Q>"
  Bus Selector2/3 -> dF1/3  "<I>"
  Bus Selector2/4 -> dF1/7, v2/1  "<ch>"
  128_shift_reg/2 -> dF1/4
  dF1/1 -> Variant Subsystem/1(valid)
  Variant Subsystem/1(valid_o) -> Bus Creator3/1  "valid"
  Bus Selector5/2 -> lfOutData/1  "<freqWord>"
  Bus Selector5/1 -> lfOutAddr/1  "<ch>"
  r_phase_delay_sel/1 -> 128_shift_reg/2
  r_feedback_limit_hi/1 -> Variant Subsystem/4(feedbackLimitHi)
  r_feedback_gain/1 -> Variant Subsystem/3(feedbackGain)
  r_feedback_polarity/1 -> Variant Subsystem/2(feedbackPolarity)
  Variant Subsystem/2(freqWordOut) -> Bus Creator3/2  "freqWord"
  Variant Subsystem/3(ch_o) -> Bus Creator3/3  "ch"
  Bus Selector6/1 -> Delay4/1  "<valid>"
  Bus Selector6/2 -> Delay5/1  "<phase>"
  BitBasher/1 -> dF1/5
  BitBasher/2 -> dF1/6
  Delay5/1 -> Reinterpret/1
  Delay4/1 -> 128_shift_reg/1  "valid"
  Reinterpret/1 -> 128_shift_reg/3  "phase"
  reset/1 -> Variant Subsystem/9(reset)
  dF1/3 -> freqWordAddr/1
  dF1/2 -> BitBasher1/1, Variant Subsystem/6(freqError)
  r_feedback_limit_lo/1 -> Variant Subsystem/5(feedbackLimitLo)
  freqWordData/1 -> Variant Subsystem/7(freqWord)
  dF1/4 -> deltaFAddr/1, Variant Subsystem/8(ch)

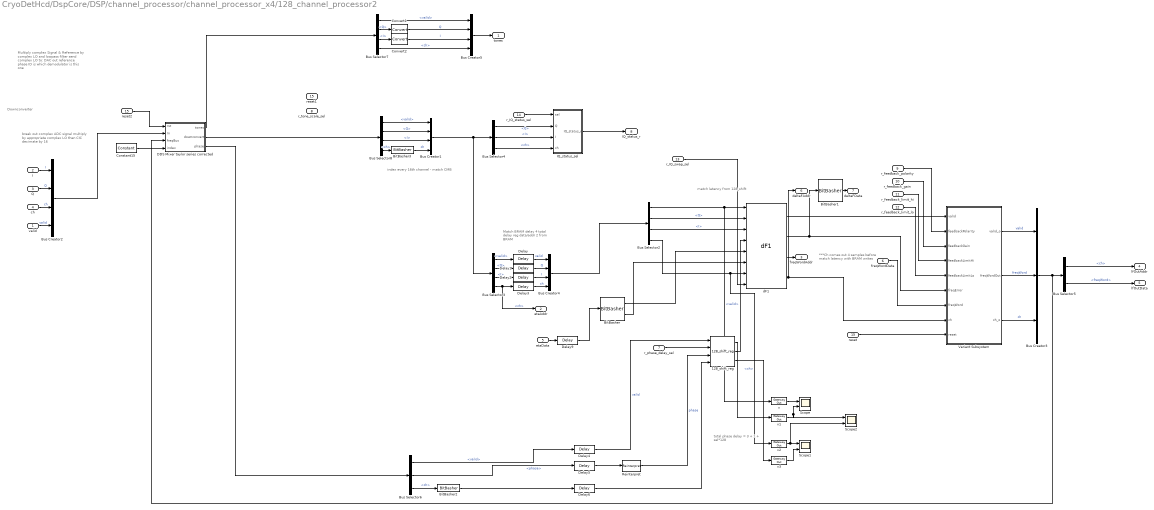
== system CryoDetHcd/DspCore/DSP/channel_processor/channel_processor_x4/128_channel_processor2 ==
  note: index every 16th channel - match CMB
  note: Downconverter
  note: Multiply complex Signal & Reference
      | by complex LO and lowpass filter
      | send complex LO to:
      | 	DAC out
      | 	reference phase
      | ID is which demodulator is this one
  note: break out complex ADC signal
      | multiply by appropriate complex LO
      | then CIC decimate by 16
  note: Match BRAM delay
      | 4 total delay
      |    reg data/addr
      |    2 from BRAM
  note: match latency from 128_shift
  note: total phase delay =
      | 3 + 1 + sel*128
  note: ***Ch comes out 4 samples before
      | match latency with BRAM writes
  valid : Inport
  I : Inport  Port=2
  Q : Inport  Port=3
  ch : Inport  Port=4
  etaData : Inport  Port=5
  freqWordData : Inport  Port=6
  r_phase_delay_sel : Inport  Port=7
  r_tone_scale_sel : Inport  Port=8
  r_feedback_polarity : Inport  Port=9
  r_feedback_gain : Inport  Port=10
  r_feedback_limit_hi : Inport  Port=11
  r_feedback_limit_lo : Inport  Port=12
  r_IQ_swap_sel : Inport  Port=13
  r_IQ_status_sel : Inport  Port=14
  reset : Inport  Port=15
  128_shift_reg : CryoDetLibCMB/128_shift_reg
  BitBasher : xbsIndex_r4/BitBasher  bitexpr=|  display_expr=off  sr_1=etaPhase  arith_type1="Signed  (2's comp)"  bin_pt1=15  sr_2=etaMag  arith_type2="Signed  (2's comp)"  bin_pt2=10  sr_3=3  arith_type3=Unsigned  bin_pt3=0  sr_4=4  arith_type4=Unsigned  bin_pt4=0  dbl_ovrd=off  block_type=bitbasher
      | etaPhase = {in[31:16]}
      | etaMag = {in[15:0]}
  BitBasher1 : xbsIndex_r4/BitBasher  bitexpr=deltaF = {8'b0, in[23:0]}  display_expr=off  sr_1=deltaF  arith_type1="Signed  (2's comp)"  bin_pt1=15  sr_2=etaMag  arith_type2="Signed  (2's comp)"  bin_pt2=10  sr_3=3  arith_type3=Unsigned  bin_pt3=0  sr_4=4  arith_type4=Unsigned  bin_pt4=0  dbl_ovrd=off  block_type=bitbasher
  BitBasher2 : xbsIndex_r4/BitBasher  bitexpr=out = {in, 4'b0000}  display_expr=off  sr_1=out  arith_type1=Unsigned  bin_pt1=0  sr_2=2  arith_type2=Unsigned  bin_pt2=0  sr_3=3  arith_type3=Unsigned  bin_pt3=0  sr_4=4  arith_type4=Unsigned  bin_pt4=0  dbl_ovrd=off  block_type=bitbasher
  BitBasher3 : xbsIndex_r4/BitBasher  bitexpr=out = {in, 4'b0000}  display_expr=off  sr_1=out  arith_type1=Unsigned  bin_pt1=0  sr_2=2  arith_type2=Unsigned  bin_pt2=0  sr_3=3  arith_type3=Unsigned  bin_pt3=0  sr_4=4  arith_type4=Unsigned  bin_pt4=0  dbl_ovrd=off  block_type=bitbasher
  Bus Creator{1..2,4..5} (4 alike) : BusCreator  Inputs=4
  Bus Creator3 : BusCreator  Inputs=3
  Bus Selector{2..3,7..8} (4 alike) : BusSelector  OutputSignals=valid,Q,I,ch
  Bus Selector4 : BusSelector  OutputSignals=Q,I,ch
  Bus Selector5 : BusSelector  OutputSignals=ch,freqWord
  Bus Selector6 : BusSelector  OutputSignals=valid,phase,ch
  Constant15 : xbsIndex_r4/Constant  const=0  gui_display_data_type=Fixed-point  arith_type=Unsigned  n_bits=4  bin_pt=0  preci_type=Single  exp_width=8  frac_width=24  explicit_period=off  period=1  equ=P=C  opselect=C  inp2=PCIN>>17  opr=+  inp1=P  carry=CIN  dbl_ovrd=off  block_type=constant
  Convert1 : xbsIndex_r4/Convert  gui_display_data_type=Fixed-point  arith_type="Signed  (2's comp)"  n_bits=16  bin_pt=15  float_type=Single  exp_bits=8  fraction_bits=24  quantization=Truncate  overflow=Wrap  en=off  latency=0  pipeline=off  dbl_ovrd=off  block_type=convert
  Convert2 : xbsIndex_r4/Convert  gui_display_data_type=Fixed-point  arith_type="Signed  (2's comp)"  n_bits=16  bin_pt=15  float_type=Single  exp_bits=8  fraction_bits=24  quantization=Truncate  overflow=Wrap  en=off  latency=0  pipeline=off  dbl_ovrd=off  block_type=convert
  DDS Mixer taylor series corrected : Subsystem  AncestorBlock=CryoDetLibCMB/DDS Mixer taylor series corrected
  Delay{,1..3} (4 alike) : xbsIndex_r4/Delay  rst=off  infoeditControl=Selection of Reset will increase slice count due to use of real FFs and instead of SRLs  en=off  latency=5  reg_retiming=off  dbl_ovrd=off  block_type=delay
  Delay{4..6,9} (4 alike) : xbsIndex_r4/Delay  rst=off  infoeditControl=Selection of Reset will increase slice count due to use of real FFs and instead of SRLs  en=off  latency=1  reg_retiming=off  dbl_ovrd=off  block_type=delay
  IQ_status_sel : Subsystem
  Reinterpret : xbsIndex_r4/Reinterpret  force_arith_type=on  arith_type="Signed  (2's comp)"  force_bin_pt=on  bin_pt=15  block_type=reinterpret
  Scope : Scope  NumInputPorts=2
  Scope1 : Scope  NumInputPorts=2
  Scope2 : Scope  NumInputPorts=2
  Variant Subsystem : Subsystem  Variant=on  OverrideUsingVariant=Variant1
  dF1 : CryoDetLibCMB/dF1
  reset1 : InportShadow  Port=15
  reset2 : InportShadow  Port=15
  v{,1..3} (4 alike) : xbsIndex_r4/Gateway Out  inherit_from_input=off  hdl_port=off  rows=1  columns=1  UseAsDAC=off  DACChannel='1'  interface=None  automatic_assignment=on  address_offset=hex2dec('00')  intf_name=''  intf_description=''  timing_constraint=None  locs_specified=off  LOCs={}  io_standard={}  block_type=gatewayout
  tones : Outport
  etaAddr : Outport  Port=2
  freqWordAddr : Outport  Port=3
  lfOutAddr : Outport  Port=4
  lfOutData : Outport  Port=5
  deltaFAddr : Outport  Port=6
  deltaFData : Outport  Port=7
  IQ_status_r : Outport  Port=8
  wires:
  dF1/4 -> Variant Subsystem/8(ch), deltaFAddr/1
  freqWordData/1 -> Variant Subsystem/7(freqWord)
  r_feedback_limit_lo/1 -> Variant Subsystem/5(feedbackLimitLo)
  dF1/2 -> Variant Subsystem/6(freqError), BitBasher1/1
  dF1/3 -> freqWordAddr/1
  reset/1 -> Variant Subsystem/9(reset)
  Reinterpret/1 -> 128_shift_reg/3  "phase"
  Delay4/1 -> 128_shift_reg/1  "valid"
  Delay5/1 -> Reinterpret/1
  BitBasher/2 -> dF1/6
  BitBasher/1 -> dF1/5
  Bus Selector6/2 -> Delay5/1  "<phase>"
  Bus Selector6/1 -> Delay4/1  "<valid>"
  Variant Subsystem/3(ch_o) -> Bus Creator3/3  "ch"
  Variant Subsystem/2(freqWordOut) -> Bus Creator3/2  "freqWord"
  r_feedback_polarity/1 -> Variant Subsystem/2(feedbackPolarity)
  r_feedback_gain/1 -> Variant Subsystem/3(feedbackGain)
  r_feedback_limit_hi/1 -> Variant Subsystem/4(feedbackLimitHi)
  r_phase_delay_sel/1 -> 128_shift_reg/2
  Bus Selector5/1 -> lfOutAddr/1  "<ch>"
  Bus Selector5/2 -> lfOutData/1  "<freqWord>"
  Variant Subsystem/1(valid_o) -> Bus Creator3/1  "valid"
  dF1/1 -> Variant Subsystem/1(valid)
  128_shift_reg/2 -> dF1/4
  Bus Selector2/4 -> v2/1, dF1/7  "<ch>"
  Bus Selector2/3 -> dF1/3  "<I>"
  Bus Selector2/2 -> dF1/2  "<Q>"
  Bus Selector2/1 -> v/1, dF1/1  "<valid>"
  Bus Creator5/1 -> tones/1
  Bus Selector7/1 -> Bus Creator5/1  "<valid>"
  Bus Selector7/4 -> Bus Creator5/4  "<ch>"
  Convert1/1 -> Bus Creator5/2  "Q"
  Convert2/1 -> Bus Creator5/3  "I"
  Bus Selector3/4 -> etaAddr/1, Delay3/1  "<ch>"
  Bus Selector3/3 -> Delay2/1  "<I>"
  Bus Selector3/2 -> Delay1/1  "<Q>"
  Bus Selector3/1 -> Delay/1  "<valid>"
  BitBasher1/1 -> deltaFData/1
  Bus Creator4/1 -> Bus Selector2/1
  etaData/1 -> Delay9/1
  Delay3/1 -> Bus Creator4/4  "ch"
  Delay2/1 -> Bus Creator4/3  "I"
  Delay1/1 -> Bus Creator4/2  "Q"
  Delay/1 -> Bus Creator4/1  "valid"
  valid/1 -> Bus Creator2/4  "valid"
  ch/1 -> Bus Creator2/3  "ch"
  Q/1 -> Bus Creator2/2  "Q"
  I/1 -> Bus Creator2/1  "I"
  DDS Mixer taylor series corrected/1(tones) -> Bus Selector7/1
  Bus Creator2/1 -> DDS Mixer taylor series corrected/2(In)
  v/1 -> Scope/1
  128_shift_reg/1 -> v1/1
  v3/1 -> Scope1/2
  128_shift_reg/3 -> v3/1
  r_IQ_swap_sel/1 -> dF1/8
  Bus Selector4/1 -> IQ_status_sel/2(Q)  "<Q>"
  Bus Selector4/2 -> IQ_status_sel/3(I)  "<I>"
  Bus Selector4/3 -> IQ_status_sel/4(ch)  "<ch>"
  r_IQ_status_sel/1 -> IQ_status_sel/1(sel)
  IQ_status_sel/1(IQ_status_r) -> IQ_status_r/1
  Delay9/1 -> BitBasher/1
  Delay6/1 -> 128_shift_reg/4
  Constant15/1 -> DDS Mixer taylor series corrected/4(index)
  reset2/1 -> DDS Mixer taylor series corrected/1(rst)
  Bus Creator3/1 -> DDS Mixer taylor series corrected/3(freqBus), Bus Selector5/1
  DDS Mixer taylor series corrected/3(phase) -> Bus Selector6/1
  Bus Selector6/3 -> BitBasher2/1  "<ch>"
  Bus Selector7/2 -> Convert1/1  "<Q>"
  Bus Selector7/3 -> Convert2/1  "<I>"
  Bus Selector8/4 -> BitBasher3/1  "<ch>"
  BitBasher3/1 -> Bus Creator1/4  "ch"
  Bus Selector8/2 -> Bus Creator1/2  "<Q>"
  Bus Selector8/1 -> Bus Creator1/1  "<valid>"
  Bus Selector8/3 -> Bus Creator1/3  "<I>"
  Bus Creator1/1 -> Bus Selector3/1, Bus Selector4/1
  DDS Mixer taylor series corrected/2(downconvert) -> Bus Selector8/1
  BitBasher2/1 -> Delay6/1
  v1/1 -> Scope2/1, Scope/2
  v2/1 -> Scope2/2, Scope1/1
